simulink model "AWES3_CL_wTether_v4_PM"  (R2022a)
settings: Solver=ode3  StartTime=0  StopTime=simInit.TSIM  FixedStep=simInit.dt  RelTol=1e-3
values from neighbouring files (symbols this model uses):
  complex_tether_flag = 1    [run_sim.m]
  Ft_max = 1870    [run_sim.m]
  q = 0    [barrier_optimization.m]
  r = 0    [barrier_optimization.m]
  random_seed = [ 24335       17059       17670        1747]    [run_sim.m]
  safety_controller = false    [run_sim.m]
  turbulence = true    [run_sim.m]
undefined symbols (not defined in the file or in its folder): aeroModel, alpha_max, alpha_min, alpha_options, base_windspeed, constr, DiscIntNeverNeededParam, dx, ENVMT, F, grid_max, grid_min, HDBK, I_table, Light, MIL, mu_max, mu_min, mu_options, P_AP2, params, SampleTime, simInit, T, u0_sim, winchParameter, x0_sim
libraries: simulink x30, aerolibwind2 x14, dspstat3 x2, pid_lib x1, aerolibwindfilters x1, aerolibcommonsys x1, matrix_library x1
(part 2 of 5)

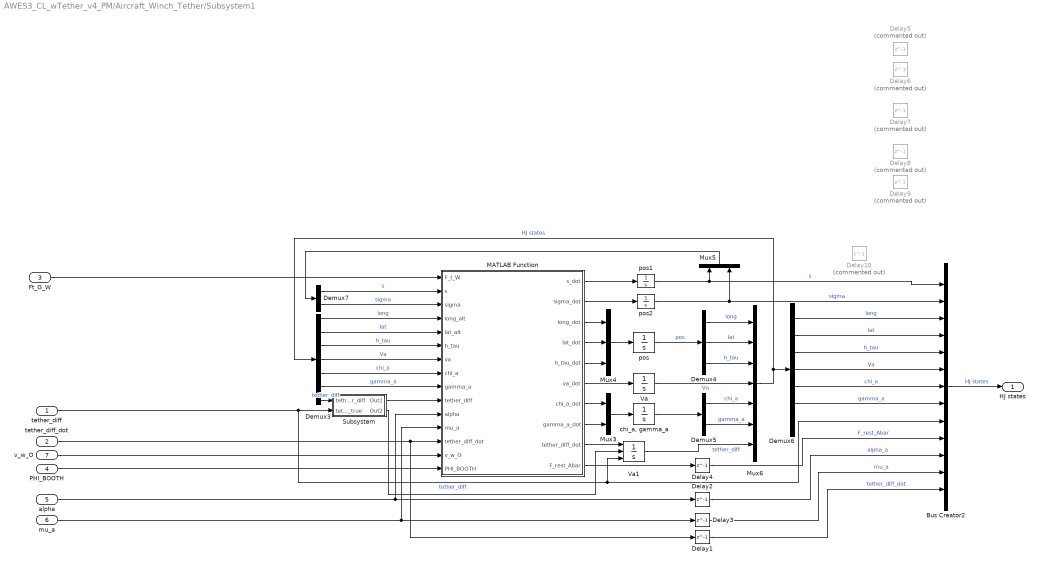
== system AWES3_CL_wTether_v4_PM/Aircraft_Winch_Tether/Subsystem1 ==
  tether_diff : Inport
  tether_diff_dot : Inport  Port=2
  Ft_G_W : Inport  Port=3
  PHI_BOOTH : Inport  Port=4
  alpha : Inport  Port=5
  mu_a : Inport  Port=6
  v_w_O : Inport  Port=7
  Bus Creator2 : BusCreator  Inputs=13
  Delay{1..4} (4 alike) : Delay  DelayLength=1  InitialCondition=0
  Delay10 : Delay  Commented=on  DelayLength=1  InitialConditionSource=Input port  InitialCondition=0
      settings: InputPortMap=u0,p4
  Delay5 : Delay  Commented=on  DelayLength=1  InitialCondition=0
  Delay6 : Delay  Commented=on  DelayLength=1  InitialCondition=0
  Delay7 : Delay  Commented=on  DelayLength=1  InitialCondition=x0_sim(10:12)
  Delay8 : Delay  Commented=on  DelayLength=1  InitialCondition=x0_sim(1)
  Delay9 : Delay  Commented=on  DelayLength=1  InitialCondition=simInit.pathangles_k_init'
  Demux3 : Demux  Outputs=7
  Demux4 : Demux  Outputs=3
  Demux5 : Demux  Outputs=2
  Demux6 : Demux  Outputs=7
  Demux7 : Demux  Outputs=2
  MATLAB Function : MATLAB Function  TreatAsAtomicUnit=on
  Mux3 : Mux  Inputs=2
  Mux4 : Mux  Inputs=3
  Mux5 : Mux  Inputs=2
  Mux6 : Mux  Inputs=7
  Subsystem : Subsystem
  Va : Integrator  InitialCondition=x0_sim(1)
  Va1 : Integrator  ExternalReset=rising  InitialConditionSource=external
  "chi_a, gamma_a" : Integrator  InitialCondition=simInit.pathangles_k_init'  WrapState=on
  pos : Integrator  InitialCondition=x0_sim(10:12)
  pos1 : Integrator  WrapState=on  WrappedStateUpperValue=2*pi  WrappedStateLowerValue=0
  pos2 : Integrator
  HJ states : Outport
  wires:
  v_w_O/1 -> MATLAB Function/14(v_w_O)
  Demux3/7 -> Subsystem/1(tether_diff)  "tether_diff"
  Subsystem/1(Out1) -> MATLAB Function/10(tether_diff)
  Delay1/1 -> Bus Creator2/13  "tether_diff_dot"
  Delay2/1 -> Bus Creator2/11  "alpha_a"
  Ft_G_W/1 -> MATLAB Function/1(F_t_W)
  MATLAB Function/9(tether_diff_dot) -> Va1/1
  Demux6/6 -> Bus Creator2/8  "gamma_a"
  Demux6/5 -> Bus Creator2/7  "chi_a"
  MATLAB Function/7(chi_a_dot) -> Mux3/1
  Demux6/2 -> Bus Creator2/4  "lat"
  Demux3/2 -> MATLAB Function/5(lat_alt)  "lat"
  MATLAB Function/4(lat_dot) -> Mux4/2
  MATLAB Function/5(h_tau_dot) -> Mux4/3
  Demux4/1 -> Mux6/1  "long"
  Demux7/2 -> MATLAB Function/3(sigma)  "sigma"
  MATLAB Function/2(sigma_dot) -> pos2/1
  MATLAB Function/8(gamma_a_dot) -> Mux3/2
  Demux3/5 -> MATLAB Function/8(chi_a)  "chi_a"
  Delay3/1 -> Bus Creator2/12  "mu_a"
  Subsystem/2(Out2) -> Va1/2
  MATLAB Function/3(long_dot) -> Mux4/1
  MATLAB Function/10(F_rest_Abar) -> Delay4/1
  Demux7/1 -> MATLAB Function/2(s)  "s"
  Mux4/1 -> pos/1
  Demux3/4 -> MATLAB Function/7(va)  "Va"
  Delay4/1 -> Bus Creator2/10  "F_rest_Abar"
  Va1/1 -> Mux6/7  "tether_diff"
  Demux3/3 -> MATLAB Function/6(h_tau)  "h_tau"
  Demux5/1 -> Mux6/5  "chi_a"
  Demux6/1 -> Bus Creator2/3  "long"
  alpha/1 -> MATLAB Function/11(alpha), Delay2/1
  MATLAB Function/1(s_dot) -> pos1/1
  MATLAB Function/6(va_dot) -> Va/1
  Demux4/2 -> Mux6/2  "lat"
  Mux3/1 -> "chi_a, gamma_a"/1
  Demux6/4 -> Bus Creator2/6  "Va"
  tether_diff_dot/1 -> Delay1/1, MATLAB Function/13("tether_diff_dot ")
  Mux6/1 -> Demux3/1, Demux6/1  "HJ states"
  PHI_BOOTH/1 -> MATLAB Function/15(PHI_BOOTH)
  Demux3/6 -> MATLAB Function/9(gamma_a)  "gamma_a"
  Demux3/1 -> MATLAB Function/4(long_alt)  "long"
  Demux4/3 -> Mux6/3  "h_tau"
  mu_a/1 -> MATLAB Function/12(mu_a), Delay3/1
  Demux6/3 -> Bus Creator2/5  "h_tau"
  pos2/1 -> Mux5/2, Bus Creator2/2  "sigma"
  Mux5/1 -> Demux7/1
  Demux5/2 -> Mux6/6  "gamma_a"
  Bus Creator2/1 -> HJ states/1  "HJ states"
  pos/1 -> Demux4/1  "pos"
  tether_diff/1 -> Bus Creator2/9, Va1/3, Subsystem/2(tether_diff_true)  "tether_diff"
  Va/1 -> Mux6/4  "Va"
  "chi_a, gamma_a"/1 -> Demux5/1
  pos1/1 -> Bus Creator2/1, Mux5/1  "s"

== system AWES3_CL_wTether_v4_PM/Aircraft_Winch_Tether/WinchDynamicsAndControl  ==
  Ft_ground_W : Inport
  Ft_set : Inport  Port=2
  retraction_flag : Inport  Port=3
  Enable : EnablePort
  Gain1 : Gain  Gain=winchParameter.radius
  Product : Product
  PureTorqueControl : Subsystem  TreatAsAtomicUnit=on
  PureTorqueControl1 : Subsystem  Commented=on
  PureTorqueControl2 : Subsystem  Commented=on  TreatAsAtomicUnit=on  SystemSampleTime=0.001
  Terminator1 : Terminator
  Transport Delay3 : TransportDelay  Commented=on  DelayTime=params.meas_delay
  Transport Delay4 : TransportDelay  Commented=on  DelayTime=params.meas_delay
  WinchDynamics : Subsystem
  l_tether : Outport  PortDimensions=1  VectorParamsAs1DForOutWhenUnconnected=off
  P_mech : Outport  Port=2  PortDimensions=1  VectorParamsAs1DForOutWhenUnconnected=off
  winch_acc : Outport  Port=3  PortDimensions=1  VectorParamsAs1DForOutWhenUnconnected=off
  v_ro : Outport  Port=4  PortDimensions=1  VectorParamsAs1DForOutWhenUnconnected=off
  wires:
  retraction_flag/1 -> PureTorqueControl/1(reset)
  WinchDynamics/4(winch_vel) -> Terminator1/1
  WinchDynamics/3(winch_acc) -> winch_acc/1  "winch_acc"
  Product/1 -> P_mech/1  "P_mech"
  Gain1/1 -> v_ro/1, Product/2
  WinchDynamics/1(tether_length) -> l_tether/1
  PureTorqueControl/1(torque_cmd) -> WinchDynamics/2(control_moments)
  Ft_ground_W/1 -> PureTorqueControl/2(F_t_m_grnd), Product/1, WinchDynamics/1(for_tether_tot)
  WinchDynamics/2(theta_dot) -> Gain1/1, PureTorqueControl/4(theta_dot)
  Ft_set/1 -> PureTorqueControl/3(F_t_set)

== system AWES3_CL_wTether_v4_PM/Aircraft_Winch_Tether/WindfieldModel ==
  Va : Inport
  pos_W : Inport  Port=2
  M_OB : Inport  Port=3
  pos_p_W : Inport  Port=4
  Clock1 : Clock
  Compare To Constant1 : simulink/Logic and Bit Operations/Compare To Constant  relop=>  const=1  OutDataTypeStr=boolean
  Constant : Constant  Value=turbulence
  Constant3 : Constant  Value=zeros(3,1)
  Constant4 : Constant  Value=ENVMT.windDirection_rad
  Delay : Delay  DelayLength=1  InitialCondition=[base_windspeed;0;0]
  Demux : Demux  Outputs=3
  Gain1 : Gain  Gain=-1
  Logical Operator : Logic  AllPortsSameDT=off  OutDataTypeStr=boolean
  MATLAB Function : MATLAB Function  TreatAsAtomicUnit=on
  MATLAB Function1 : MATLAB Function  TreatAsAtomicUnit=on
  Product : Product  Multiplication=Matrix(*)
  Reshape : Reshape  OutputDimensionality=Column vector (2-D)
  Reshape1 : Reshape  OutputDimensionality=Column vector (2-D)
  Saturation : Saturate  UpperLimit=inf  LowerLimit=10
  Selector : Selector  InputPortWidth=3  IndexOptions=Index vector (dialog)  Indices=3  OutputSizes=1
  Selector3 : Selector  InputPortWidth=3*T.np  IndexOptions=Index vector (dialog)  Indices=3:3:3*T.np  OutputSizes=1
  ShearWind : Subsystem  TreatAsAtomicUnit=on  mask{Wdeg=ENVMT.windDirection_rad*180/pi}
      mask prompts: Wdeg "Windirection"
      settings: MinAlgLoopOccurrences=on
  Subsystem1 : Subsystem
  Sum : Sum  Inputs=|++
  Switch : Switch  Criteria=u2 > Threshold  SaturateOnIntegerOverflow=off  InputSameDT=off
  Switch1 : Switch  Criteria=u2 > Threshold  SaturateOnIntegerOverflow=off  InputSameDT=off
  Terminator : Terminator
  To Workspace6 : ToWorkspace  Commented=on  VariableName=v_x_w_W  SaveFormat=Timeseries  SampleTime=0.1
  Windshear : Subsystem  TreatAsAtomicUnit=on
      settings: MinAlgLoopOccurrences=on
  turbulence bounds : Scope  NumInputPorts=3
  v_w_W : Outport  VectorParamsAs1DForOutWhenUnconnected=off
  v_w_O : Outport  Port=2  VectorParamsAs1DForOutWhenUnconnected=off
  v_w_p : Outport  Port=3  VectorParamsAs1DForOutWhenUnconnected=off
  wires:
  MATLAB Function/1(vec_W) -> Reshape1/1, To Workspace6/1
  Product/1 -> MATLAB Function/2(vec_O)
  M_OB/1 -> Subsystem1/2(DCM), Product/1, Windshear/1(DCM)
  Windshear/1(V_shear_mDs) -> Gain1/1
  Gain1/1 -> Product/2
  pos_p_W/1 -> Selector3/1
  Subsystem1/1(v_w_turb_W_noDelay) -> Switch/1
  Constant4/1 -> MATLAB Function/1(wind_direction_rad), MATLAB Function1/1(wind_direction_rad)
  Sum/1 -> Delay/1
  Va/1 -> Saturation/1
  Clock1/1 -> Compare To Constant1/1
  Switch/1 -> Demux/1, Sum/2
  Constant3/1 -> Reshape/1
  Reshape/1 -> Switch/3, Switch1/3
  Selector3/1 -> ShearWind/1(Altitude_p_vec)
  ShearWind/1(v_w_p) -> v_w_p/1
  Reshape1/1 -> Sum/1
  Selector/1 -> Subsystem1/1(h), Windshear/2(altitude)
  pos_W/1 -> Selector/1
  Saturation/1 -> Subsystem1/3(Va)
  Subsystem1/2(w0_turbulence_B) -> Switch1/1
  Delay/1 -> v_w_W/1, MATLAB Function1/2(vec_W)
  Switch1/1 -> Terminator/1
  MATLAB Function1/1(vec_O) -> v_w_O/1
  Logical Operator/1 -> Switch1/2, Switch/2
  Compare To Constant1/1 -> Logical Operator/1
  Constant/1 -> Logical Operator/2
  Demux/1 -> turbulence bounds/1  "u_{g,W}"
  Demux/2 -> turbulence bounds/2  "v_{g,W}"
  Demux/3 -> turbulence bounds/3  "w_{g,W}"

== system AWES3_CL_wTether_v4_PM/Aircraft_Winch_Tether/norm ==
  Ft_G_W : Inport
  Dot Product : DotProduct  OutDataTypeStr=Inherit: Inherit via internal rule
  Sqrt : Sqrt
  F_t_m : Outport
  wires:
  Sqrt/1 -> F_t_m/1
  Dot Product/1 -> Sqrt/1
  Ft_G_W/1 -> Dot Product/2, Dot Product/1

== system AWES3_CL_wTether_v4_PM/Aircraft_Winch_Tether/norm2 ==
  <pos_G_W_m> : Inport
  Dot Product1 : DotProduct  OutDataTypeStr=Inherit: Inherit via internal rule
  Sqrt1 : Sqrt
  Out1 : Outport
  wires:
  Sqrt1/1 -> Out1/1
  <pos_G_W_m>/1 -> Dot Product1/1, Dot Product1/2
  Dot Product1/1 -> Sqrt1/1

== system AWES3_CL_wTether_v4_PM/FlightController/Logic ==
  mode : Inport
  Compare To Constant : simulink/Logic and Bit Operations/Compare To Constant  relop===  const=5  OutDataTypeStr=boolean
  Compare To Constant1 : simulink/Logic and Bit Operations/Compare To Constant  relop===  const=6  OutDataTypeStr=boolean
  Compare To Constant2 : simulink/Logic and Bit Operations/Compare To Constant  relop===  const=4  OutDataTypeStr=boolean
  Compare To Constant7 : simulink/Logic and Bit Operations/Compare To Constant  relop===  const=7  OutDataTypeStr=boolean
  Logical Operator : Logic  Operator=OR  AllPortsSameDT=off  OutDataTypeStr=boolean
  Logical Operator1 : Logic  Operator=OR  AllPortsSameDT=off  OutDataTypeStr=boolean
  fm45 : Outport  VectorParamsAs1DForOutWhenUnconnected=off
  fm5 : Outport  Port=2  VectorParamsAs1DForOutWhenUnconnected=off
  fm67 : Outport  Port=3  VectorParamsAs1DForOutWhenUnconnected=off
  wires:
  mode/1 -> Compare To Constant1/1, Compare To Constant7/1, Compare To Constant2/1, Compare To Constant/1
  Compare To Constant2/1 -> Logical Operator/2
  Compare To Constant/1 -> fm5/1, Logical Operator/1
  Compare To Constant7/1 -> Logical Operator1/1
  Logical Operator/1 -> fm45/1
  Compare To Constant1/1 -> Logical Operator1/2
  Logical Operator1/1 -> fm67/1

== system AWES3_CL_wTether_v4_PM/FlightController/Retraction ==
  Ft_set : Inport
  F_t_m : Inport  Port=2
  phi0_retraction : Inport  Port=3
  v_w_O : Inport  Port=4
  AirframeOutput_Bus : Inport  Port=5
  Enable : EnablePort  StatesWhenEnabling=reset
  Bus Selector : BusSelector  OutputSignals=airdata,vel_K_O_mDs,pos_G_O_m,pathAngles_a
  CalculateAttitudeCmds : Subsystem  TreatAsAtomicUnit=on  SystemSampleTime=0.01
  Gain : Gain  Gain=params.w0_mu_a_emulation
  Gain1 : Gain  Gain=params.w0_alpha_a_emulation
  GuidanceFlatEarth : Subsystem
  Integrator : Integrator  InitialConditionSource=external
  Integrator2 : Integrator  InitialConditionSource=external
  Selector3 : Selector  InputPortWidth=2  IndexOptions=Index vector (dialog)  Indices=2  OutputSizes=1
  Selector4 : Selector  InputPortWidth=3  IndexOptions=Index vector (dialog)  Indices=1  OutputSizes=1
  Sum2 : Sum  Inputs=|+-
  Sum4 : Sum  Inputs=|+-
  transition_flag : Outport  VectorParamsAs1DForOutWhenUnconnected=off
  approachFlag : Outport  Port=2  VectorParamsAs1DForOutWhenUnconnected=off
  retraction_error : Outport  Port=3  VectorParamsAs1DForOutWhenUnconnected=off
  path_cmd : Outport  Port=4  VectorParamsAs1DForOutWhenUnconnected=off
  mu_a_c : Outport  Port=5  VectorParamsAs1DForOutWhenUnconnected=off
  alpha_a_c : Outport  Port=6  VectorParamsAs1DForOutWhenUnconnected=off
  target_W : Outport  Port=7  VectorParamsAs1DForOutWhenUnconnected=off
  wires:
  Ft_set/1 -> CalculateAttitudeCmds/2(Ft_set)
  F_t_m/1 -> CalculateAttitudeCmds/3(F_t_m)
  GuidanceFlatEarth/2(course_path) -> Selector3/1, CalculateAttitudeCmds/1(pathangles_k_cmd)
  phi0_retraction/1 -> GuidanceFlatEarth/3(phi0_retraction)
  v_w_O/1 -> CalculateAttitudeCmds/5(v_w_O)
  GuidanceFlatEarth/3(transition_flag) -> transition_flag/1
  Gain/1 -> Integrator/1
  Sum2/1 -> Gain/1
  Sum4/1 -> Gain1/1
  Gain1/1 -> Integrator2/1
  GuidanceFlatEarth/1(approachFlag) -> approachFlag/1
  CalculateAttitudeCmds/1(mu_a_cmd) -> Integrator/2, Sum2/1
  Integrator2/1 -> alpha_a_c/1, Sum4/2
  CalculateAttitudeCmds/2(alpha_cmd) -> Integrator2/2, Sum4/1
  Selector4/1 -> GuidanceFlatEarth/4(Va)  "Va"
  AirframeOutput_Bus/1 -> Bus Selector/1
  Bus Selector/1 -> CalculateAttitudeCmds/4(airdata), Selector4/1  "<airdata>"
  Bus Selector/2 -> CalculateAttitudeCmds/6(v_k_O), GuidanceFlatEarth/2("vel_K_O ")  "<vel_K_O_mDs>"
  Bus Selector/3 -> GuidanceFlatEarth/1(pos_G_O), CalculateAttitudeCmds/7(p_G_O)  "<pos_G_O_m>"
  Bus Selector/4 -> CalculateAttitudeCmds/8(pathangles_a)  "<pathAngles_a>"
  GuidanceFlatEarth/5(retraction_path_error) -> retraction_error/1
  Selector3/1 -> path_cmd/1
  Integrator/1 -> mu_a_c/1, Sum2/2
  GuidanceFlatEarth/6(target_W) -> target_W/1

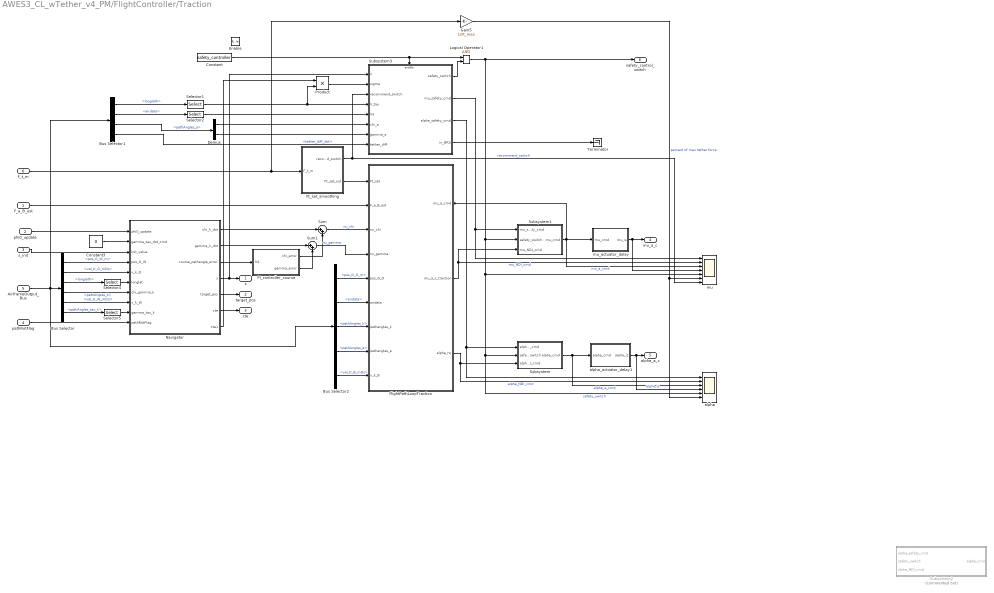
== system AWES3_CL_wTether_v4_PM/FlightController/Traction ==
  F_a_B_est : Inport  PortDimensions=[3,1]
  phi0_update : Inport  Port=2
  s_init : Inport  Port=3
  pathRotFlag : Inport  Port=4
  AirframeOutput_Bus : Inport  Port=5
  F_t_m : Inport  Port=6
  Enable : EnablePort  StatesWhenEnabling=reset
  Bus Selector : BusSelector  OutputSignals=pos_G_W_m,vel_K_O_mDs,longlath,pathAngles_k,vel_K_W_mDs,pathAngles_tau_k
  Bus Selector1 : BusSelector  OutputSignals=longlath,airdata,pathAngles_a,tether_diff_dot
  Bus Selector2 : BusSelector  OutputSignals=pos_G_O_m,airdata,pathAngles_k,pathAngles_a,vel_K_B_mDs
  Constant : Constant  Value=safety_controller
  Constant3 : Constant  Value=0
  Demux : Demux  Outputs=2
  FlightPathLoopTraction : Subsystem  TreatAsAtomicUnit=on  SystemSampleTime=0.01
      settings: PortSchema="{\"entries\":[{\"content\":{\"sides\":[{\"content\":{\"connectorIds\":[\"In1\",\"In2\",\"In3\",\"In4\",\"In5\",\"In6\",\"In7\",\"In8\",\"In9\"]},\"type\":\"ConnectorPlacement.EquallySpacedRectSide\",\"uuid\":\"b7109311-1544-44fe-bd69-1e2e43ab6b67\"},{\"content\":{\"connectorIds\":[\"In10\",\"Out1\",\"Out2\"],\"side\":\"RIGHT\"},\"type\":\"ConnectorPlacement.EquallySpacedRectSide\",\"uuid\":\"c8951929-38d2-4cb1-8810-0230a107c88f\"},{\"content\":{\"connectorIds\":[],\"side\":\"TOP\"},\"type\":\"ConnectorPlacement.EquallySpacedRectSide\",\"uuid\":\"6d80cd61-d04a-45e7-94c9-cced10ffbec4\"},{\"content\":{\"connectorIds\":[],\"side\":\"BOTTOM\"},\"type\":\"ConnectorPlacement.EquallySpacedRectSide\",\"uuid\":\"866676a3-b2d6-41a1-a2bd-8e289d291c77\"}]},\"type\":\"ConnectorPlacement.EquallySpacedConnector\",\"uuid\":\"d3b31c18-1533-41c6-b15d-746d0974b403\"}],\"packageUris\":[\"http://schema.mathworks.com/mf0/Connector/R2020b\"],\"version\":\"1.0\"}"
  Ft_set_smoothing : Subsystem
  Gain5 : Gain  Gain=1/Ft_max
  Logical Operator1 : Logic  IconShape=distinctive  AllPortsSameDT=off  OutDataTypeStr=boolean
  Navigator : Subsystem
  PI_controller_course : Subsystem
  Product : Product
  Selector1 : Selector  InputPortWidth=3  IndexOptions=Index vector (dialog)  Indices=3  OutputSizes=1
  Selector2 : Selector  InputPortWidth=3  IndexOptions=Index vector (dialog)  Indices=1  OutputSizes=1
  Selector4 : Selector  InputPortWidth=3  IndexOptions=Index vector (dialog)  Indices=1:2  OutputSizes=1
  Selector5 : Selector  InputPortWidth=2  IndexOptions=Index vector (dialog)  Indices=2  OutputSizes=1
  Subsystem : Subsystem
  Subsystem1 : Subsystem
  Subsystem2 : Subsystem  Commented=on
  Subsystem3 : Subsystem
  Sum : Sum  Inputs=|++
  Sum1 : Sum  Inputs=|++
  Terminator : Terminator
  alpha : Scope  NumInputPorts=6
  alpha_actuator_delay1 : Subsystem
  mu : Scope  NumInputPorts=7
  mu_actuator_delay : Subsystem
  s : Outport  VectorParamsAs1DForOutWhenUnconnected=off
  target_pos : Outport  Port=2  VectorParamsAs1DForOutWhenUnconnected=off
  cte : Outport  Port=3  VectorParamsAs1DForOutWhenUnconnected=off
  mu_a_c : Outport  Port=4  VectorParamsAs1DForOutWhenUnconnected=off
  alpha_a_c : Outport  Port=5  VectorParamsAs1DForOutWhenUnconnected=off
  safety_control_switch : Outport  Port=6
  wires:
  F_a_B_est/1 -> FlightPathLoopTraction/2(F_a_B_est)
  Constant3/1 -> Navigator/2(gamma_tau_dot_cmd)
  Navigator/1(chi_k_dot) -> Sum/1
  Navigator/2(gamma_k_dot) -> Sum1/1
  s_init/1 -> Navigator/3(init_value)
  Sum1/1 -> FlightPathLoopTraction/4(nu_gamma)  "nu_gamma"
  Sum/1 -> FlightPathLoopTraction/3(nu_chi)  "nu_chi"
  Selector4/1 -> Navigator/6(longlat)
  Selector5/1 -> Navigator/9(gamma_tau_k)
  phi0_update/1 -> Navigator/1(phi0_update)
  Subsystem/1(alpha_cmd) -> alpha_actuator_delay1/1(alpha_cmd), alpha/3  "alpha_a_cmd"
  pathRotFlag/1 -> Navigator/10(pathRotFlag)
  Navigator/5(target_pos) -> target_pos/1
  Bus Selector/4 -> Navigator/7(chi_gamma_k)  "<pathAngles_k>"
  Bus Selector/3 -> Selector4/1  "<longlath>"
  Bus Selector/6 -> Selector5/1  "<pathAngles_tau_k>"
  Bus Selector/2 -> Navigator/5(v_k_O)  "<vel_K_O_mDs>"
  Bus Selector/1 -> Navigator/4(pos_G_W)  "<pos_G_W_m>"
  Bus Selector/5 -> Navigator/8(v_k_W)  "<vel_K_W_mDs>"
  Bus Selector2/1 -> FlightPathLoopTraction/5(pos_G_O)  "<pos_G_O_m>"
  Bus Selector2/2 -> FlightPathLoopTraction/6(airdata)  "<airdata>"
  Bus Selector2/3 -> FlightPathLoopTraction/7(pathangles_k)  "<pathAngles_k>"
  Bus Selector2/4 -> FlightPathLoopTraction/8(pathangles_a)  "<pathAngles_a>"
  Bus Selector2/5 -> FlightPathLoopTraction/9(v_k_B)  "<vel_K_B_mDs>"
  AirframeOutput_Bus/1 -> Bus Selector1/1, Bus Selector2/1, Bus Selector/1
  Navigator/4(s) -> Subsystem3/1(s), s/1
  alpha_actuator_delay1/1(alpha_is) -> alpha_a_c/1, alpha/4  "alpha_is"
  Gain5/1 -> alpha/6, mu/6  "percent of max tether force"
  FlightPathLoopTraction/2(alpha_rq) -> Subsystem/3(alpha_NDI_cmd), alpha/2  "alpha_NDI_cmd"
  Subsystem1/1(mu_cmd) -> FlightPathLoopTraction/10(mu_a_cmd), mu_actuator_delay/1(mu_cmd), mu/3  "mu_a_cmd"
  FlightPathLoopTraction/1(mu_a_c_traction) -> Subsystem1/3(mu_NDI_cmd), mu/2  "mu_NDI_cmd"
  Logical Operator1/1 -> Subsystem1/2(safety_switch), Subsystem/2(safety_switch), alpha/5, mu/5, safety_control_switch/1  "safety_switch"
  Subsystem3/2(mu_safety_cmd) -> Subsystem1/1(mu_safety_cmd), mu/1
  Subsystem3/4(in_BRS) -> Terminator/1
  F_t_m/1 -> Gain5/1, Ft_set_smoothing/1(F_t_m)
  Ft_set_smoothing/2(Ft_set_out) -> FlightPathLoopTraction/1(Ft_set)
  Ft_set_smoothing/1(recommend_switch) -> Subsystem3/3(recommend_switch), mu/7  "recommend_switch"
  mu_actuator_delay/1(mu_is) -> mu_a_c/1, mu/4
  Navigator/3("course_pathangle_error ") -> PI_controller_course/1(In1)
  PI_controller_course/1(chi_error) -> Sum/2
  PI_controller_course/2(gamma_error) -> Sum1/2
  Constant/1 -> Subsystem3/Enable, Logical Operator1/1
  Subsystem3/1(safety_switch) -> Logical Operator1/2
  Selector1/1 -> Subsystem3/4(h_tau), Product/2
  Bus Selector1/1 -> Selector1/1  "<longlath>"
  Bus Selector1/2 -> Selector2/1  "<airdata>"
  Selector2/1 -> Subsystem3/5(Va)
  Demux/2 -> Subsystem3/7(gamma_a)
  Bus Selector1/3 -> Demux/1  "<pathAngles_a>"
  Demux/1 -> Subsystem3/6(chi_a)
  Bus Selector1/4 -> Subsystem3/8(tether_diff)  "<tether_diff_dot>"
  Navigator/6(cte) -> cte/1
  Product/1 -> Subsystem3/2(sigma)
  Navigator/7(cte1) -> Product/1
  Subsystem3/3(alpha_safety_cmd) -> Subsystem/1(alpha_safety_cmd), alpha/1

== system AWES3_CL_wTether_v4_PM/HighLevelControlSystem/Subsystem1 ==
  x0 : Inport
  SetPoint : Inport  Port=2
  airspeed : Inport  Port=3
  mode : Inport  Port=4
  avoid : Inport  Port=5
  Compare To Constant : simulink/Logic and Bit Operations/Compare To Constant  relop=>  const=params.vamax  OutDataTypeStr=boolean
  Compare To Constant1 : simulink/Logic and Bit Operations/Compare To Constant  relop===  const=7  OutDataTypeStr=boolean
  Constant : Constant  Value=params.Ft_set_retraction
  Constant1 : Constant  Value=0
  HighWindGain1 : Gain  Gain=w0^2
  HighWindGain2 : Gain  Gain=2*w0
  Integrator : Integrator  ExternalReset=rising
  Integrator1 : Integrator  ExternalReset=rising  InitialConditionSource=external
  Logical Operator : Logic  AllPortsSameDT=off  OutDataTypeStr=boolean
  Logical Operator1 : Logic  Operator=NOT  AllPortsSameDT=off  OutDataTypeStr=boolean
  Logical Operator2 : Logic  Operator=OR  AllPortsSameDT=off  OutDataTypeStr=boolean
  Sum1 : Sum  Inputs=|+-
  Sum2 : Sum  Inputs=|+-
  Switch1 : Switch  Criteria=u2 > Threshold  SaturateOnIntegerOverflow=off  InputSameDT=off
  Switch2 : Switch  Criteria=u2 > Threshold  SaturateOnIntegerOverflow=off  InputSameDT=off
  Switch3 : Switch  Criteria=u2 > Threshold  SaturateOnIntegerOverflow=off  InputSameDT=off
  SetPoint_Filtered : Outport  VectorParamsAs1DForOutWhenUnconnected=off
  wires:
  x0/1 -> Integrator1/3
  Integrator1/1 -> Switch2/3, Sum2/2
  HighWindGain1/1 -> Sum1/1
  Sum2/1 -> HighWindGain1/1
  Integrator/1 -> HighWindGain2/1, Switch3/3
  HighWindGain2/1 -> Sum1/2
  Sum1/1 -> Switch1/3
  Logical Operator/1 -> Switch3/2, Switch2/2, Switch1/2
  mode/1 -> Compare To Constant1/1
  Constant/1 -> Switch2/1
  SetPoint/1 -> Sum2/1
  Switch2/1 -> SetPoint_Filtered/1
  Switch1/1 -> Integrator/1
  Switch3/1 -> Integrator1/1
  Constant1/1 -> Switch1/1, Switch3/1
  airspeed/1 -> Compare To Constant/1
  Compare To Constant/1 -> Logical Operator/1
  Compare To Constant1/1 -> Logical Operator/2, Logical Operator2/1
  avoid/1 -> Logical Operator1/1
  Logical Operator1/1 -> Logical Operator2/2
  Logical Operator2/1 -> Integrator1/2, Integrator/2

== system AWES3_CL_wTether_v4_PM/HighLevelControlSystem/Subsystem2 ==
  mode : Inport
  Compare To Constant : simulink/Logic and Bit Operations/Compare To Constant  relop===  const=6  OutDataTypeStr=boolean
  Compare To Constant8 : simulink/Logic and Bit Operations/Compare To Constant  relop===  const=7  OutDataTypeStr=boolean
  Logical Operator1 : Logic  Operator=OR  AllPortsSameDT=off  OutDataTypeStr=boolean
  retraction_flag : Outport  VectorParamsAs1DForOutWhenUnconnected=off
  wires:
  Compare To Constant/1 -> Logical Operator1/2
  mode/1 -> Compare To Constant8/1, Compare To Constant/1
  Compare To Constant8/1 -> Logical Operator1/1
  Logical Operator1/1 -> retraction_flag/1

== system AWES3_CL_wTether_v4_PM/HighLevelControlSystem/Subsystem4 ==
  mode : Inport
  avoid_flag : Inport  Port=2
  Compare To Constant : simulink/Logic and Bit Operations/Compare To Constant  relop===  const=6  OutDataTypeStr=boolean
  Compare To Constant8 : simulink/Logic and Bit Operations/Compare To Constant  relop===  const=4  OutDataTypeStr=boolean
  Logical Operator : Logic  Operator=NOT  Inputs=3  AllPortsSameDT=off  OutDataTypeStr=boolean
  Logical Operator1 : Logic  Operator=NOT  Inputs=3  AllPortsSameDT=off  OutDataTypeStr=boolean
  Logical Operator2 : Logic  Inputs=3  AllPortsSameDT=off  OutDataTypeStr=boolean
  Logical Operator4 : Logic  Operator=NOT  Inputs=3  AllPortsSameDT=off  OutDataTypeStr=boolean
  Out1 : Outport  VectorParamsAs1DForOutWhenUnconnected=off
  wires:
  Compare To Constant8/1 -> Logical Operator1/1
  mode/1 -> Compare To Constant/1, Compare To Constant8/1
  Compare To Constant/1 -> Logical Operator4/1
  avoid_flag/1 -> Logical Operator/1
  Logical Operator/1 -> Logical Operator2/3
  Logical Operator2/1 -> Out1/1
  Logical Operator4/1 -> Logical Operator2/2
  Logical Operator1/1 -> Logical Operator2/1

== system AWES3_CL_wTether_v4_PM/Visualization/Tether Rupture1 ==
  In1 : Inport
  Constant3 : Constant  Value=Ft_max
  Delay : Delay  DelayLength=1  InitialCondition=0
  Relational Operator2 : RelationalOperator  Operator=>  OutDataTypeStr=boolean  RndMeth=Simplest  InputSameDT=off
  Stop Simulation : Stop
  wires:
  In1/1 -> Relational Operator2/1
  Constant3/1 -> Relational Operator2/2
  Relational Operator2/1 -> Delay/1
  Delay/1 -> Stop Simulation/1

== system AWES3_CL_wTether_v4_PM/Visualization/Tether Rupture2 ==
  In1 : Inport
  Constant3 : Constant  Value=Ft_max
  Delay : Delay  DelayLength=1  InitialCondition=0
  Relational Operator2 : RelationalOperator  Operator=>  OutDataTypeStr=boolean  RndMeth=Simplest  InputSameDT=off
  Stop Simulation : Stop
  To Workspace25 : ToWorkspace  VariableName=rupture  SaveFormat=Timeseries  SampleTime=-1
      settings: MaxDataPoints=1
  wires:
  In1/1 -> Relational Operator2/1
  Constant3/1 -> Relational Operator2/2
  Relational Operator2/1 -> To Workspace25/1, Delay/1
  Delay/1 -> Stop Simulation/1

== system AWES3_CL_wTether_v4_PM/Visualization/hold max ==
  In1 : Inport
  Delay : Delay  DelayLength=1  InitialCondition=0
  Max : MinMax  Function=max  Inputs=2
  Out1 : Outport
  wires:
  Max/1 -> Out1/1, Delay/1
  Delay/1 -> Max/2
  In1/1 -> Max/1

== system AWES3_CL_wTether_v4_PM/Aircraft_Winch_Tether/ParticleTetherModel/Plot tether_diff_dot ==
  tether_diff_dot_is : Inport
  Constant3 : Constant  Value=0
  Delay : Delay  DelayLength=1  InitialCondition=0
  Delay1 : Delay  DelayLength=1  InitialCondition=0  SampleTime=0.5
  Delay2 : Delay  DelayLength=1  InitialCondition=0  SampleTime=0.25
  Interval Test : simulink/Logic and Bit Operations/Interval Test  IntervalClosedRight=on  uplimit=0.005  IntervalClosedLeft=on  lowlimit=-0.005  OutDataTypeStr=boolean
  Logical Operator1 : Logic  Inputs=3  AllPortsSameDT=off  OutDataTypeStr=boolean
  Logical Operator2 : Logic  Operator=OR  AllPortsSameDT=off  OutDataTypeStr=boolean
  Switch4 : Switch  Criteria=u2 > Threshold  SaturateOnIntegerOverflow=off  InputSameDT=off
  tether_diff_dot : Scope
  wires:
  Switch4/1 -> tether_diff_dot/1
  Constant3/1 -> Switch4/3
  tether_diff_dot_is/1 -> Switch4/1, Interval Test/1
  Interval Test/1 -> Delay2/1, Delay1/1, Logical Operator1/1
  Delay2/1 -> Logical Operator1/2
  Logical Operator2/1 -> Delay/1, Switch4/2
  Delay1/1 -> Logical Operator1/3
  Logical Operator1/1 -> Logical Operator2/1
  Delay/1 -> Logical Operator2/2

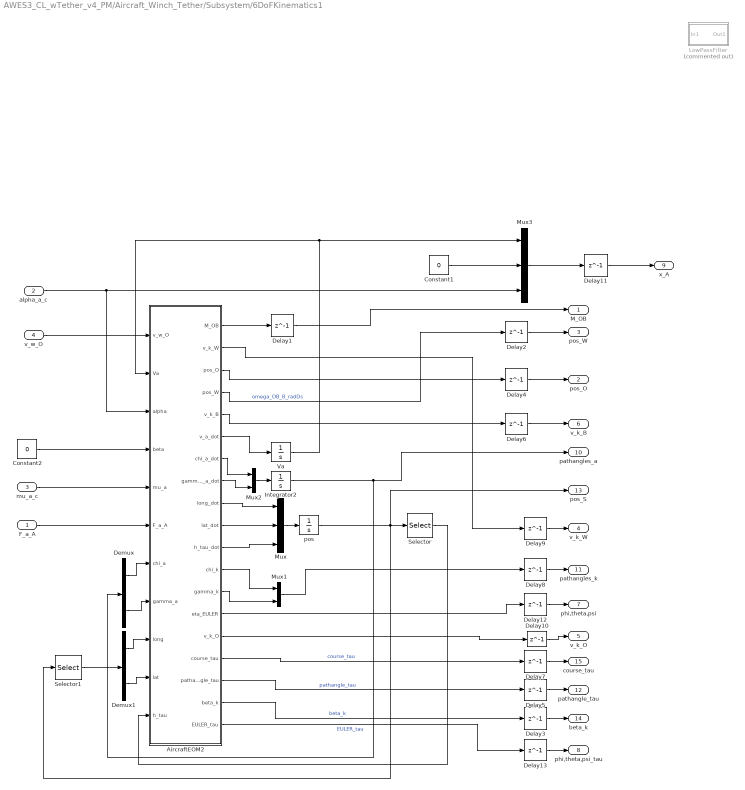
== system AWES3_CL_wTether_v4_PM/Aircraft_Winch_Tether/Subsystem/6DoFKinematics1 ==
  F_a_A : Inport
  alpha_a_c : Inport  Port=2
  mu_a_c : Inport  Port=3
  v_w_O : Inport  Port=4
  AircraftEOM2 : MATLAB Function  TreatAsAtomicUnit=on
  Constant1 : Constant  Value=0
  Constant2 : Constant  Value=0
  Delay1 : Delay  DelayLength=1  InitialCondition=simInit.M_OB
  Delay10 : Delay  DelayLength=1  InitialCondition=simInit.v_k_O_init
  Delay11 : Delay  DelayLength=1  InitialCondition=x0_sim(1:3)
  Delay12 : Delay  DelayLength=1  InitialCondition=simInit.EULER_init
  Delay13 : Delay  DelayLength=1  InitialCondition=x0_sim(4:6)
  Delay2 : Delay  DelayLength=1  InitialCondition=simInit.pos_W_init
  Delay3 : Delay  DelayLength=1
  Delay4 : Delay  DelayLength=1  InitialCondition=simInit.pos_O_init'
  Delay5 : Delay  DelayLength=1  InitialCondition=zeros(2,1)
  Delay6 : Delay  DelayLength=1  InitialCondition=simInit.v_k_B_init
  Delay7 : Delay  DelayLength=1
  Delay8 : Delay  DelayLength=1  InitialCondition=simInit.pathangles_k_init
  Delay9 : Delay  DelayLength=1  InitialCondition=simInit.v_k_W_init
  Demux : Demux  Outputs=2
  Demux1 : Demux  Outputs=2
  Integrator2 : Integrator  InitialCondition=simInit.pathangles_k_init'  WrapState=on
  LowPassFilter : Subsystem  Commented=on  mask{w0=100, zeta=1, x0=x0_sim(1)}
  Mux : Mux  Inputs=3
  Mux1 : Mux  Inputs=2
  Mux2 : Mux  Inputs=2
  Mux3 : Mux  Inputs=3
  Selector : Selector  InputPortWidth=3  IndexOptions=Index vector (dialog)  Indices=3  OutputSizes=1
  Selector1 : Selector  InputPortWidth=3  IndexOptions=Index vector (dialog)  Indices=1:2  OutputSizes=1
  Va : Integrator  InitialCondition=x0_sim(1)
  pos : Integrator  InitialCondition=x0_sim(10:12)
  M_OB : Outport  VectorParamsAs1DForOutWhenUnconnected=off
  pos_O : Outport  Port=2  VectorParamsAs1DForOutWhenUnconnected=off
  pos_W : Outport  Port=3  VectorParamsAs1DForOutWhenUnconnected=off
  v_k_W : Outport  Port=4  VectorParamsAs1DForOutWhenUnconnected=off
  v_k_O : Outport  Port=5  VectorParamsAs1DForOutWhenUnconnected=off
  v_k_B : Outport  Port=6  VectorParamsAs1DForOutWhenUnconnected=off
  phi,theta,psi : Outport  Port=7  VectorParamsAs1DForOutWhenUnconnected=off
  phi,theta,psi_tau : Outport  Port=8  VectorParamsAs1DForOutWhenUnconnected=off
  x_A : Outport  Port=9  VectorParamsAs1DForOutWhenUnconnected=off
  pathangles_a : Outport  Port=10  VectorParamsAs1DForOutWhenUnconnected=off
  pathangles_k : Outport  Port=11  VectorParamsAs1DForOutWhenUnconnected=off
  pathangle_tau : Outport  Port=12  VectorParamsAs1DForOutWhenUnconnected=off
  pos_S : Outport  Port=13  VectorParamsAs1DForOutWhenUnconnected=off
  beta_k : Outport  Port=14  VectorParamsAs1DForOutWhenUnconnected=off
  course_tau : Outport  Port=15  VectorParamsAs1DForOutWhenUnconnected=off
  wires:
  Delay12/1 -> phi,theta,psi/1
  v_w_O/1 -> AircraftEOM2/1(v_w_O)
  Delay11/1 -> x_A/1
  Delay6/1 -> v_k_B/1
  Delay4/1 -> pos_O/1
  Delay2/1 -> pos_W/1
  Selector1/1 -> Demux1/1
  AircraftEOM2/19(EULER_tau) -> Delay13/1  "EULER_tau"
  AircraftEOM2/18(beta_k) -> Delay3/1  "beta_k"
  AircraftEOM2/17(pathangle_tau) -> Delay5/1  "pathangle_tau"
  AircraftEOM2/16(course_tau) -> Delay7/1  "course_tau"
  AircraftEOM2/5(v_k_B) -> Delay6/1
  AircraftEOM2/4(pos_W) -> Delay2/1  "omega_OB_B_radDs"
  Demux1/2 -> AircraftEOM2/10(lat)
  Demux1/1 -> AircraftEOM2/9(long)
  Selector/1 -> AircraftEOM2/11(h_tau)
  AircraftEOM2/11(h_tau_dot) -> Mux/3
  Demux/1 -> AircraftEOM2/7(chi_a)
  Demux/2 -> AircraftEOM2/8(gamma_a)
  Constant2/1 -> AircraftEOM2/4(beta)
  alpha_a_c/1 -> AircraftEOM2/3(alpha), Mux3/3
  Constant1/1 -> Mux3/2
  Mux2/1 -> Integrator2/1
  AircraftEOM2/8(gamma_a_dot) -> Mux2/2
  AircraftEOM2/7(chi_a_dot) -> Mux2/1
  AircraftEOM2/6(v_a_dot) -> Va/1
  AircraftEOM2/2(v_k_W) -> Delay9/1
  AircraftEOM2/15(v_k_O) -> Delay10/1
  Mux1/1 -> Delay8/1
  AircraftEOM2/13(gamma_k) -> Mux1/2
  AircraftEOM2/12(chi_k) -> Mux1/1
  AircraftEOM2/10(lat_dot) -> Mux/2
  AircraftEOM2/9(long_dot) -> Mux/1
  Mux/1 -> pos/1
  AircraftEOM2/1(M_OB) -> Delay1/1
  Mux3/1 -> Delay11/1
  Delay13/1 -> phi,theta,psi_tau/1
  Delay10/1 -> v_k_O/1
  Delay9/1 -> v_k_W/1
  Delay8/1 -> pathangles_k/1
  Delay7/1 -> course_tau/1
  Delay5/1 -> pathangle_tau/1
  Delay3/1 -> beta_k/1
  AircraftEOM2/3(pos_O) -> Delay4/1
  mu_a_c/1 -> AircraftEOM2/5(mu_a)
  F_a_A/1 -> AircraftEOM2/6(F_a_A)
  AircraftEOM2/14(eta_EULER) -> Delay12/1
  Delay1/1 -> M_OB/1
  Integrator2/1 -> Demux/1, pathangles_a/1
  Va/1 -> AircraftEOM2/2(Va), Mux3/1
  pos/1 -> Selector1/1, Selector/1, pos_S/1

== system AWES3_CL_wTether_v4_PM/Aircraft_Winch_Tether/Subsystem1/Subsystem ==
  tether_diff : Inport
  tether_diff_true : Inport  Port=2
  Compare To Zero : simulink/Logic and Bit Operations/Compare To Zero  relop=>  OutDataTypeStr=boolean
  Delay5 : Delay  InitialCondition=0
  Max : MinMax  Function=max  Inputs=2  OutDataTypeStr=boolean
  Switch3 : Switch  Criteria=u2 > Threshold  SaturateOnIntegerOverflow=off  InputSameDT=off
  Out1 : Outport
  Out2 : Outport  Port=2
  wires:
  tether_diff/1 -> Switch3/1
  Compare To Zero/1 -> Max/2
  Switch3/1 -> Out1/1
  Delay5/1 -> Max/1, Switch3/2, Out2/1
  tether_diff_true/1 -> Switch3/3, Compare To Zero/1
  Max/1 -> Delay5/1

== system AWES3_CL_wTether_v4_PM/Aircraft_Winch_Tether/WinchDynamicsAndControl /PureTorqueControl ==
  reset : Inport
  F_t_m_grnd : Inport  Port=2
  F_t_set : Inport  Port=3
  theta_dot : Inport  Port=4
  Constant4 : Constant  Value=constr.winchParameter.a_max/winchParameter.radius
  Constant5 : Constant  Value=constr.winchParameter.a_min/winchParameter.radius
  Gain : Gain  Gain=winchParameter.inertia
  Gain10 : Gain  Gain=winchParameter.friction
  Gain3 : Gain  Gain=winchParameter.radius
  Gain4 : Gain  Gain=winchParameter.inertia
  PI-ForceController : Subsystem
  Saturation Dynamic : simulink/Discontinuities/Saturation Dynamic  OutMin=[]  OutMax=[]  OutDataTypeStr=Inherit: Same as second input  OutDataType=fixdt(1, 16)  OutScaling=2^-10  DoSatur=off
  Subsystem : Subsystem
  Sum : Sum  Inputs=|-++
  Sum3 : Sum  Inputs=|-++
  Sum6 : Sum  Inputs=+-|
  Sum7 : Sum  Inputs=+-|
  torque_cmd : Outport  VectorParamsAs1DForOutWhenUnconnected=off
  wires:
  F_t_set/1 -> Sum6/2  "d"
  Gain3/1 -> Sum/1, Sum3/1
  Constant4/1 -> Gain/1
  Gain/1 -> Sum/2
  Sum/1 -> Saturation Dynamic/1
  Constant5/1 -> Gain4/1
  Gain4/1 -> Sum3/2
  Sum3/1 -> Saturation Dynamic/3
  Gain10/1 -> Sum/3, Sum3/3
  reset/1 -> PI-ForceController/2(retraction)
  Sum7/1 -> PI-ForceController/3(controlDeficitDue2Sat)
  Sum6/1 -> PI-ForceController/4(e_Ft)
  F_t_m_grnd/1 -> Sum6/1, Gain3/1  "F_t_m"
  theta_dot/1 -> Gain10/1  "F_t_m"
  PI-ForceController/1(TorqueCmd) -> PI-ForceController/1(preSat), Saturation Dynamic/2, Sum7/1  "F_t_m"
  Saturation Dynamic/1 -> Subsystem/1(In1), Sum7/2  "F_t_m"
  Subsystem/1(Out1) -> torque_cmd/1  "F_t_m"

== system AWES3_CL_wTether_v4_PM/Aircraft_Winch_Tether/WinchDynamicsAndControl /PureTorqueControl1 ==
  retraction_flag : Inport
  F_t_m_grnd : Inport  Port=2
  F_t_set : Inport  Port=3
  theta_dot : Inport  Port=4
  Constant : Constant  Value=0
  Constant4 : Constant  Value=constr.winchParameter.a_max/winchParameter.radius
  Constant5 : Constant  Value=constr.winchParameter.a_min/winchParameter.radius
  Dot Product1 : DotProduct  OutDataTypeStr=Inherit: Inherit via internal rule
  Gain : Gain  Gain=winchParameter.inertia
  Gain10 : Gain  Gain=winchParameter.friction
  Gain3 : Gain  Gain=winchParameter.radius
  Gain4 : Gain  Gain=winchParameter.inertia
  Gain5 : Gain  Gain=winchParameter.inertia/(winchParameter.radius*P_AP2.mass)
  Gain6 : Gain  Gain=winchParameter.radius
  PI-ForceController : Subsystem
  Rate Transition : RateTransition  OutPortSampleTime=0.001
  Saturation Dynamic : simulink/Discontinuities/Saturation Dynamic  OutMin=[]  OutMax=[]  OutDataTypeStr=Inherit: Same as second input  OutDataType=fixdt(1, 16)  OutScaling=2^-10  DoSatur=off
  Sqrt1 : Sqrt
  Sum : Sum  Inputs=|-++
  Sum1 : Sum  Inputs=|++
  Sum3 : Sum  Inputs=|-++
  Sum4 : Sum  Inputs=+-
  Sum5 : Sum  Inputs=|+-
  Sum6 : Sum  Inputs=+-|
  Sum7 : Sum  Inputs=-+|
  Terminator : Terminator
  torque_cmd : Outport  VectorParamsAs1DForOutWhenUnconnected=off
  wires:
  PI-ForceController/1(TorqueCmd) -> Sum1/2
  Sum6/1 -> PI-ForceController/3(e_Ft)
  Sum7/1 -> PI-ForceController/2(controlDeficitDue2Sat)
  retraction_flag/1 -> PI-ForceController/1(RetractionFlag)
  Constant/1 -> Sum1/1
  theta_dot/1 -> Gain10/1
  Rate Transition/1 -> torque_cmd/1
  F_t_m_grnd/1 -> Gain3/1, Gain6/1, Dot Product1/2, Dot Product1/1
  Dot Product1/1 -> Sqrt1/1
  Sum4/1 -> Terminator/1
  Sum5/1 -> Gain5/1
  Gain5/1 -> Sum4/1
  Gain6/1 -> Sum4/2
  Sqrt1/1 -> Sum5/1, Sum6/1
  Saturation Dynamic/1 -> Rate Transition/1, Sum7/2
  Gain10/1 -> Sum3/3, Sum/3
  Sum1/1 -> Sum7/1, Saturation Dynamic/2
  Sum3/1 -> Saturation Dynamic/3
  Gain4/1 -> Sum3/2
  Constant5/1 -> Gain4/1
  Sum/1 -> Saturation Dynamic/1
  Gain/1 -> Sum/2
  Constant4/1 -> Gain/1
  Gain3/1 -> Sum3/1, Sum/1
  F_t_set/1 -> Sum6/2, Sum5/2  "d"

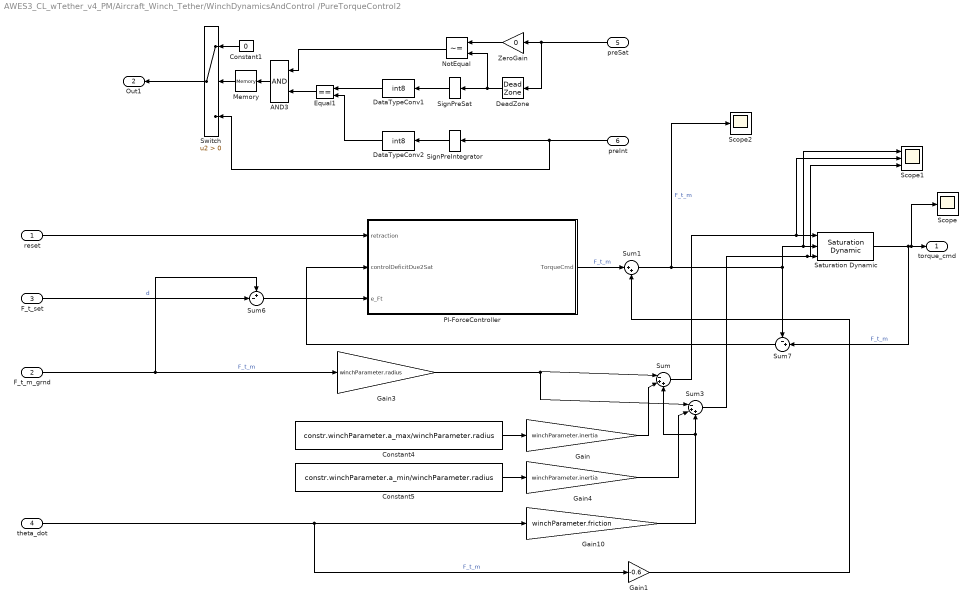
== system AWES3_CL_wTether_v4_PM/Aircraft_Winch_Tether/WinchDynamicsAndControl /PureTorqueControl2 ==
  reset : Inport
  F_t_m_grnd : Inport  Port=2
  F_t_set : Inport  Port=3
  theta_dot : Inport  Port=4
  preSat : Inport  Port=5  SampleTime=SampleTime
  preInt : Inport  Port=6  SampleTime=SampleTime
  AND3 : Logic  DisableCoverage=on  OutDataTypeStr=boolean
  Constant1 : Constant  DisableCoverage=on  Value=0  OutDataTypeStr=Inherit: Inherit via back propagation  PreserveConstantTs=on
  Constant4 : Constant  Value=constr.winchParameter.a_max/winchParameter.radius
  Constant5 : Constant  Value=constr.winchParameter.a_min/winchParameter.radius
  DataTypeConv1 : DataTypeConversion  DisableCoverage=on  OutDataTypeStr=int8  SaturateOnIntegerOverflow=off  RndMeth=Floor
  DataTypeConv2 : DataTypeConversion  DisableCoverage=on  OutDataTypeStr=int8  SaturateOnIntegerOverflow=off  RndMeth=Floor
  DeadZone : DeadZone  DisableCoverage=on  LowerValue=LowerSaturationLimit  UpperValue=UpperSaturationLimit  SaturateOnIntegerOverflow=off
  Equal1 : RelationalOperator  DisableCoverage=on  Operator===  OutDataTypeStr=boolean  RndMeth=Floor  InputSameDT=off
  Gain : Gain  Gain=winchParameter.inertia
  Gain1 : Gain  Gain=-0.6
  Gain10 : Gain  Gain=winchParameter.friction
  Gain3 : Gain  Gain=winchParameter.radius
  Gain4 : Gain  Gain=winchParameter.inertia
  Memory : Memory  DisableCoverage=on  InheritSampleTime=on
  NotEqual : RelationalOperator  DisableCoverage=on  Operator=~=  OutDataTypeStr=boolean  RndMeth=Floor  InputSameDT=off
  PI-ForceController : Subsystem
  Saturation Dynamic : simulink/Discontinuities/Saturation Dynamic  OutMin=[]  OutMax=[]  OutDataTypeStr=Inherit: Same as second input  OutDataType=fixdt(1, 16)  OutScaling=2^-10  DoSatur=off
  Scope : Scope
  Scope1 : Scope  NumInputPorts=3
  Scope2 : Scope
  SignPreIntegrator : Signum  DisableCoverage=on
  SignPreSat : Signum  DisableCoverage=on
  Sum : Sum  Inputs=|-++
  Sum1 : Sum  Inputs=|++
  Sum3 : Sum  Inputs=|-++
  Sum6 : Sum  Inputs=+-|
  Sum7 : Sum  Inputs=-+|
  Switch : Switch  Criteria=u2 > Threshold  SaturateOnIntegerOverflow=off
  ZeroGain : Gain  DisableCoverage=on  Gain=0  OutDataTypeStr=Inherit: Same as input  ParamDataTypeStr=Inherit: Same as input
  torque_cmd : Outport  VectorParamsAs1DForOutWhenUnconnected=off
  Out1 : Outport  Port=2  SampleTime=SampleTime  VectorParamsAs1DForOutWhenUnconnected=off
  wires:
  Switch/1 -> Out1/1
  preSat/1 -> ZeroGain/1, DeadZone/1
  Memory/1 -> Switch/2
  SignPreIntegrator/1 -> DataTypeConv2/1
  ZeroGain/1 -> NotEqual/1
  NotEqual/1 -> AND3/1
  SignPreSat/1 -> DataTypeConv1/1
  preInt/1 -> SignPreIntegrator/1, Switch/3
  Constant1/1 -> Switch/1
  AND3/1 -> Memory/1
  DeadZone/1 -> SignPreSat/1, NotEqual/2
  DataTypeConv2/1 -> Equal1/2
  DataTypeConv1/1 -> Equal1/1
  Equal1/1 -> AND3/2
  Gain1/1 -> Sum1/2
  PI-ForceController/1(TorqueCmd) -> Sum1/1  "F_t_m"
  Saturation Dynamic/1 -> Sum7/2, torque_cmd/1, Scope/1  "F_t_m"
  Sum1/1 -> Sum7/1, Saturation Dynamic/2, Scope1/1, Scope2/1  "F_t_m"
  theta_dot/1 -> Gain10/1, Gain1/1  "F_t_m"
  F_t_m_grnd/1 -> Gain3/1, Sum6/1  "F_t_m"
  Sum6/1 -> PI-ForceController/3(e_Ft)
  Sum7/1 -> PI-ForceController/2(controlDeficitDue2Sat)
  reset/1 -> PI-ForceController/1(retraction)
  Gain10/1 -> Sum3/3, Sum/3
  Sum3/1 -> Saturation Dynamic/3, Scope1/3
  Gain4/1 -> Sum3/2
  Constant5/1 -> Gain4/1
  Sum/1 -> Saturation Dynamic/1, Scope1/2
  Gain/1 -> Sum/2
  Constant4/1 -> Gain/1
  Gain3/1 -> Sum3/1, Sum/1
  F_t_set/1 -> Sum6/2  "d"

== system AWES3_CL_wTether_v4_PM/Aircraft_Winch_Tether/WinchDynamicsAndControl /WinchDynamics ==
  for_tether_tot : Inport
  control_moments : Inport  Port=2
  Discrete-Time Integrator1 : DiscreteIntegrator  InitialCondition=simInit.winch_angle_init  SampleTime=simInit.dt  ICPrevOutput=DiscIntNeverNeededParam  ICPrevScaledInput=DiscIntNeverNeededParam
  Discrete-Time Integrator3 : DiscreteIntegrator  SampleTime=simInit.dt  LimitOutput=on  UpperSaturationLimit=constr.winchParameter.v_max/winchParameter.radius  LowerSaturationLimit=constr.winchParameter.v_min/winchParameter.radius  ICPrevOutput=DiscIntNeverNeededParam  ICPrevScaledInput=DiscIntNeverNeededParam
  FrictionCoefficient : Gain  Gain=winchParameter.friction
  Gain{,2..4} (4 alike) : Gain  Gain=winchParameter.radius
  Gain1 : Gain  Gain=1/winchParameter.inertia
  Saturation1 : Saturate  UpperLimit=constr.winchParameter.a_max/winchParameter.radius  LowerLimit=constr.winchParameter.a_min/winchParameter.radius
  Sum : Sum  Inputs=+-+
  tether_length : Outport  VectorParamsAs1DForOutWhenUnconnected=off
  theta_dot : Outport  Port=2  VectorParamsAs1DForOutWhenUnconnected=off
  winch_acc : Outport  Port=3  VectorParamsAs1DForOutWhenUnconnected=off
  winch_vel : Outport  Port=4  VectorParamsAs1DForOutWhenUnconnected=off
  wires:
  Gain/1 -> tether_length/1
  Gain2/1 -> Sum/1
  Sum/1 -> Gain1/1
  Discrete-Time Integrator1/1 -> Gain/1  "winch_angle"
  Discrete-Time Integrator3/1 -> Gain4/1, Discrete-Time Integrator1/1, theta_dot/1, FrictionCoefficient/1  "winch_angVel"
  control_moments/1 -> Sum/3
  FrictionCoefficient/1 -> Sum/2
  for_tether_tot/1 -> Gain2/1
  Gain1/1 -> Saturation1/1
  Saturation1/1 -> Gain3/1, Discrete-Time Integrator3/1  "omega_dot"
  Gain4/1 -> winch_vel/1
  Gain3/1 -> winch_acc/1

== system AWES3_CL_wTether_v4_PM/Aircraft_Winch_Tether/WindfieldModel/ShearWind ==
  Altitude_p_vec : Inport  Unit=m
  3ft-->inf : Saturate  UpperLimit=inf  LowerLimit=3
  Length Conversion : aerolibwind2/Wind Shear Model/Length Conversion  SystemSampleTime=-1  VariantActivationTime=update diagram  Latency=0  AutoFrameSizeCalculation=off
      settings: SourceProductBaseCode=AE
  MATLAB Function : MATLAB Function  TreatAsAtomicUnit=on
  Product : Product  Inputs=*/  InputSameDT=on  SaturateOnIntegerOverflow=on  OutDataTypeStr=Inherit: Same as first input
  Product1 : Product  InputSameDT=on  SaturateOnIntegerOverflow=on  OutDataTypeStr=Inherit: Same as first input
  Reshape : Reshape  OutputDimensionality=Column vector (2-D)
  Wdeg2 : Constant  Value=base_windspeed  OutDataTypeStr=Inherit: Inherit via back propagation
  h/z0 : Gain  Gain=1/0.15  SaturateOnIntegerOverflow=on  OutDataTypeStr=Inherit: Same as input  ParamDataTypeStr=Inherit: Same as input
  ln(h/z0) : Math  Operator=log  SignedPower=on
  ln(ref_height/z0) : Math  Operator=log  SignedPower=on
  ref_height/z0 : Constant  Value=20/0.15  OutDataTypeStr=Inherit: Inherit via back propagation
  v_w_p : Outport  Unit=m/s  VectorParamsAs1DForOutWhenUnconnected=off
  wires:
  3ft-->inf/1 -> h/z0/1
  Product/1 -> Product1/1
  Wdeg2/1 -> Product1/2
  ref_height/z0/1 -> ln(ref_height/z0)/1
  h/z0/1 -> ln(h/z0)/1
  ln(ref_height/z0)/1 -> Product/2
  Reshape/1 -> MATLAB Function/1(v_w_u)
  ln(h/z0)/1 -> Product/1
  Product1/1 -> Reshape/1
  Length Conversion/1 -> 3ft-->inf/1
  MATLAB Function/1(v_w_p_mat) -> v_w_p/1
  Altitude_p_vec/1 -> Length Conversion/1

== system AWES3_CL_wTether_v4_PM/Aircraft_Winch_Tether/WindfieldModel/Subsystem1 ==
  h : Inport
  DCM : Inport  Port=2
  Va : Inport  Port=3
  Constant1 : Constant  Commented=on  Value=ENVMT.windDirection_rad
  Constant2 : Constant  Commented=on  Value=ENVMT.windDirection_rad
  Constant3 : Constant  Value=ENVMT.windDirection_rad
  Dryden Wind Turbulence Model (Continuous (+q +r)) : aerolibwind2/Dryden Wind Turbulence Model  (Continuous (+q -r))  units=Metric (MKS)  spec=MIL-HDBK-1797B  model=Continuous Dryden (+q +r)  W20=base_windspeed  Wdeg=ENVMT.windDirection_rad*180/pi  TurbProb=2x10^-1  L_high=533.4  Wingspan=P_AP2.b  ts=0.1  Seed=random_seed  T_on=on
  Dryden Wind Turbulence Model (Discrete (+q +r)) : aerolibwind2/Dryden Wind Turbulence Model  (Continuous (+q -r))  Commented=on  units=Metric (MKS)  spec=MIL-F-8785C  model=Discrete Dryden (+q +r)  W20=base_windspeed  Wdeg=ENVMT.windDirection_rad*180/pi  TurbProb=10^-2 - Light  L_high=533.4  Wingspan=P_AP2.b  ts=0.1  Seed=random_seed  T_on=on
  MATLAB Function : MATLAB Function  Commented=on  TreatAsAtomicUnit=on
  MATLAB Function1 : MATLAB Function  Commented=on  TreatAsAtomicUnit=on
  MATLAB Function2 : MATLAB Function  TreatAsAtomicUnit=on
  Product : Product  Commented=on  Multiplication=Matrix(*)
  Product1 : Product  Commented=on  Multiplication=Matrix(*)
  Product2 : Product  Multiplication=Matrix(*)
  Reshape : Reshape  Commented=on  OutputDimensionality=Column vector (2-D)
  Reshape1 : Reshape  Commented=on  OutputDimensionality=Column vector (2-D)
  Reshape2 : Reshape  OutputDimensionality=Column vector (2-D)
  Subsystem : Subsystem  Commented=on  mask{W20=base_windspeed, Wdeg=ENVMT.windDirection_rad*180/pi, L_high=533.4, TurbProb=1, dt=0.1, Wingspan=P_AP2.b, T_on=on}
      mask prompts: W20 "Wind speed at 6m:"; Wdeg "Wind direction at 6m:"; L_high "Scale length at medium/high altitude (m):"; TurbProb "Probability of exceedance of high-altitude intensity:"; dt "Sampling time:"; T_on "Turbulence on:"
      mask init:
      | h_vec = [.5 1.75 3.75 7.5 15 25 35 45 55 65 75 80]*1000;% feet
      | sigma_vec(1,:) = [3.2 2.2 1.5 zeros(1,9)]; % ft/sec
      | sigma_vec(2,:) = [4.2 3.6 3.3 1.6 zeros(1,8)];
      | sigma_vec(3,:) = [6.6 6.9 7.4 6.7 4.6 2.7 0.4 zeros(1,5)];
      | sigma_vec(4,:) = [8.6 9.6 10.6 10.1 8.0 6.6 5.0 4.2 2.7 zeros(1,3)];
      | sigma_vec(5,:) = [11.8 13.0 16.0 15.1 11.6 9.7 8.1 8.2 7.9 4.9 3.2 2.1];
      | sigma_vec(6,:) = [15.6 17.6 23.0 23.6 22.1 20.0 16.0 15.1 12.1 7.9 6.2 5.1];
      | sigma_vec(7,:) = [18.7 21.5 28.4 30.2 30.7 31.0 25.2 23.1 17.5 10.7 8.4 7.2];
      | max_height_low = 1000;
      | %min_height_high = 2000;
      | min_height_high = 1750;
  Transpose1 : Math  Operator=transpose  SignedPower=on
  v_w_turb_W_noDelay : Outport  VectorParamsAs1DForOutWhenUnconnected=off
  w0_turbulence_B : Outport  Port=2  VectorParamsAs1DForOutWhenUnconnected=off
  wires:
  h/1 -> Dryden Wind Turbulence Model (Continuous (+q +r))/1, Dryden Wind Turbulence Model (Discrete (+q +r))/1, Subsystem/1(Altitude)
  Va/1 -> Dryden Wind Turbulence Model (Continuous (+q +r))/2, Dryden Wind Turbulence Model (Discrete (+q +r))/2, Subsystem/2(Airspeed)
  Subsystem/1(ug,vg,wg) -> Product/2
  Product/1 -> Reshape/1
  Constant1/1 -> MATLAB Function/2(windDir)
  Transpose1/1 -> Dryden Wind Turbulence Model (Continuous (+q +r))/3, Dryden Wind Turbulence Model (Discrete (+q +r))/3, Subsystem/3(DCM)
  Subsystem/2(pg,qg,rg) -> w0_turbulence_B/1
  Reshape/1 -> MATLAB Function/1(u)
  Reshape1/1 -> MATLAB Function1/1(u)
  Constant2/1 -> MATLAB Function1/2(windDir)
  Product1/1 -> Reshape1/1
  Dryden Wind Turbulence Model (Discrete (+q +r))/1 -> Product1/2
  Product2/1 -> Reshape2/1
  Reshape2/1 -> MATLAB Function2/1(u)
  Dryden Wind Turbulence Model (Continuous (+q +r))/1 -> Product2/2
  DCM/1 -> Product/1, Product2/1, Product1/1, Transpose1/1
  Constant3/1 -> MATLAB Function2/2(windDir)
  MATLAB Function2/1(y) -> v_w_turb_W_noDelay/1

== system AWES3_CL_wTether_v4_PM/Aircraft_Winch_Tether/WindfieldModel/Windshear ==
  DCM : Inport
  altitude : Inport  Port=2
  Math Function : Math  Operator=transpose  SignedPower=on
  Wind Shear Model : aerolibwind2/Wind Shear Model  units=Metric (MKS)  phase=Category C - Terminal Flight Phase  W_20=base_windspeed  Wdeg=ENVMT.windDirection_rad*180/pi
  V_shear_mDs : Outport  VectorParamsAs1DForOutWhenUnconnected=off
  wires:
  altitude/1 -> Wind Shear Model/1
  DCM/1 -> Math Function/1
  Math Function/1 -> Wind Shear Model/2
  Wind Shear Model/1 -> V_shear_mDs/1
